simulink library "components_lib"  (Simulink 6.2)
undefined symbols (not defined in the file): A_ang_c, A_att_c, A_est, A_kalman, albedo_onboard_wrapper, B_ang_c, B_att_c, B_est, B_kalman, C_ang_c, C_att_c, C_est, C_i, C_kalman, C_p, Cd, D_ang_c, D_att_c, D_est, D_kalman, Dim, DiscIntNeverNeededParam, Hr, Hs, inerti, Ki, Kr, Ks, magnitude, otoquest, otoquest_with_pro, qmethod, rho, sat_temp_start, ss_proj3, sun_emu_angles2currents, sun_emu_vec2angles, Ts, vector_projection_onto_plane, w_mw_i, w_mw_init, zenith2ref
libraries: components_lib x163, simulink x44, albedo_lib x4, Accessories_lib x3, simulink_extras x2, discrete_bdot_filter x1
(part 1 of 5)
settings Model: Creator=jdgr01  LastModifiedBy=Martin  ExtModeAutoUpdateStatusClock=off

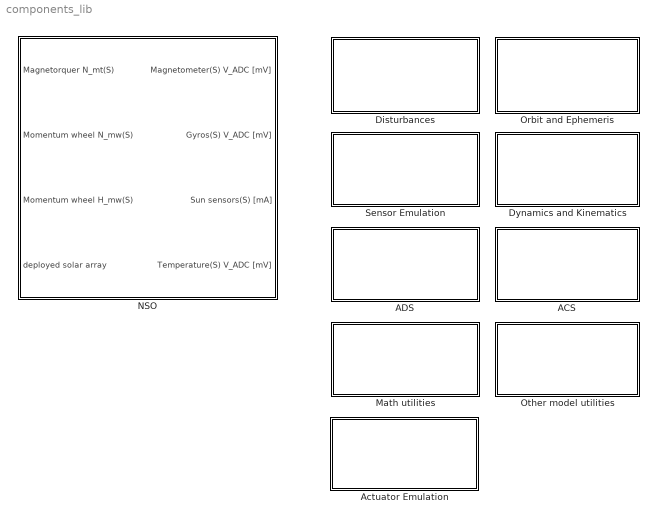
== system components_lib ==
  ACS : Subsystem
  ADS : Subsystem
  Actuator Emulation : Subsystem
  Disturbances : Subsystem
  Dynamics and Kinematics : Subsystem
  Math utilities : Subsystem
  NSO : Subsystem  Tag=AAUSAT-II Model  Description=AAUSAT-II Model  mask{r_com_s=[0.05 0.05 0.15], sat_temp_start=0, r_com_s_deployed=[0.05 0.05 0.125], mass_sc=3, Dim=[0.1 0.1 0.3], inertia_c=[25 25 5]/1e3, inertia_d=[42.3 42.3 28.4]/1e3, init_jd=2452315.56, q_s_c=[0 0 0 1], q_init_s_i=[sqrt(0.5) 0 0 sqrt(0.5)], w_init_s=[0.1 0.1 0.1]*0, Cd=2, rho=9.25e-13, enable_sensor_emulation=off, alb_emu_enabled=off, enable_dist=off}
      mask prompts: r_com_s "Center of mass (S)"; sat_temp_start "Start temperature of satellite [K]"; r_com_s_deployed "Center of mass (deployed)"; mass_sc "Mass of spacecraft (kg)"; Dim "Dimensions of the satellite (m)"; inertia_c "Folded inertia matrix(C)"; inertia_d "Deployed inertia matrix(C)"; init_jd "Initial time (JD)"; q_s_c "Controller reference frame (S->C)"; q_init_s_i "Initial attitude q_i(S->I)"; w_init_s "Initial angular rate W(S)"; Cd "Drag Coefficient"; rho "Air Density"; enable_sensor_emulation "Enable sensor emulation?"; alb_emu_enabled "Enable albedo emulation?"; enable_dist "Enable disturbances"
      mask Display:
      | image(imread('NSO.jpg'));
      | color('r');
      | port_label('input', 1, 'N_mt(S)');
      | port_label('input', 2, 'N_mw(S)');
      | port_label('input', 3, 'H_mw(S)');
      | port_label('input', 4, 'Deployed solar array');
      | port_label('output', 1, 'Magnetometer(S) V_ADC [mV]');
      | port_label('output', 2, 'Gyros(S) V_ADC [mV]');
      | port_label('output', 3, 'Sun sensors(S) [mA]');
      | port_label('output', 4, 'Temperature(S) V_ADC [mV]');
  Orbit and Ephemeris : Subsystem
  Other model utilities : Subsystem
  Sensor Emulation : Subsystem

== system components_lib/ACS ==
  Controllers : Subsystem
  Magnetorquer power driver : Subsystem
  magnetorquer driver : Subsystem
      mask Display:
      | port_label('output',1,'I_out')
      | port_label('input',1,'Nmt(sat)')
      | port_label('input',2,'B(sat)')

== system components_lib/ADS ==
  Attitude Determination : Subsystem
  FDI : Subsystem
  On-board model : Subsystem

== system components_lib/Actuator Emulation ==
  Magnetorquer : Subsystem  mask{v_max_mt=5, coil_dim=[0.07 0.21], L_mt=26.956e-3, n_mt=435, A_wire_mt=(pi/4)*0.0002^2, sigma_0_mt=1.7e-8, alpha_0_mt=3.9e-3, T_0_mt=293}
      mask prompts: v_max_mt "Maximum voltage"; coil_dim "Coil dimensions [x y]"; L_mt "Coil inductance"; n_mt "Coil winding number"; A_wire_mt "Wire cross sectional area"; sigma_0_mt "Wire resistivity"; alpha_0_mt "Wire resistivity temp. coef."; T_0_mt "Wire resistivity base temp."
  Magnetorquer without L : Subsystem  mask{v_max_mt=5, coil_dim=[0.07 0.21], n_mt=435, A_wire_mt=(pi/4)*0.0002^2, sigma_0_mt=1.7e-8, alpha_0_mt=3.9e-3, T_0_mt=293}
      mask prompts: v_max_mt "Maximum voltage"; coil_dim "Coil dimensions [x y]"; n_mt "Coil winding number"; A_wire_mt "Wire cross sectional area"; sigma_0_mt "Wire resistivity"; alpha_0_mt "Wire resistivity temp. coef."; T_0_mt "Wire resistivity base temp."
  Momentum wheel : Subsystem  mask{v_max_mw=3, v_min_mw=0, R_mw=8, L_mw=0.07e-3, C_t=2.67e-3, C_s=0.0027, mu_f=39.606e-9, I_mw=4.139e-6}
      mask prompts: v_max_mw "Maximum voltage"; v_min_mw "Minimum voltage"; R_mw "Amature resistance"; L_mw "Amature inductance"; C_t "Motor torque constant"; C_s "Motor speed constant"; mu_f "Viscous friction coef."; I_mw "Momentum wheel inertia"
  NSO magnetorquers : Subsystem
  NSO magnetorquers without L : Subsystem
  NSO momentum wheels : Subsystem  mask{w_mw_i=[1078.6 1078.6 1078.6] *0.5}
      mask prompts: w_mw_i "Initial Angular Velocity"
  NSO mw HW : Subsystem  mask{C_p=0.4, C_i=0.04, w_mw_init=w_mw_i(1)}
      mask prompts: C_p "Motor controller p-gain"; C_i "Motor controller i-gain"; w_mw_init "Initial Angular velocity"
  PI-controller : Subsystem  mask{PI_cp=C_p, PI_ci=C_i, int_limit_max=3, int_limit_min=-3}
      mask prompts: PI_cp "Porpotional gain"; PI_ci "Integrator gain"; int_limit_max "Integrator limit max"; int_limit_min "Integrator limit min"

== system components_lib/Disturbances ==
  Atmospheric : Subsystem
  Disturbances : Subsystem
  Exposed area : Subsystem  mask{dim_sat_area=Dim, dim_sat_array=[-0.30,-0.30]}
      mask prompts: dim_sat_area "Satellite Body Dimentions [x,y,z]"; dim_sat_array "Solar Array Dimentions [array1_y,array2_x]"
  Gravity : Subsystem  mask{G=6.673e-11, M_sun=1.98892e30, M_moon=7.36e22, M_earth=5.9742e24}
      mask prompts: G "Gravitational Constant (m^3/kgs^2)"; M_sun "Mass of the Sun (kg)"; M_moon "Mass of the Moon (kg)"; M_earth "Mass of the Earth (kg)"
  Magnetic residual disturbance : Subsystem
  Radiation (I) : Subsystem

== system components_lib/Dynamics and Kinematics ==
  Spacecraft Dynamics : Subsystem

== system components_lib/Math utilities ==
  Quaternion operations : Subsystem
  Vector operations : Subsystem

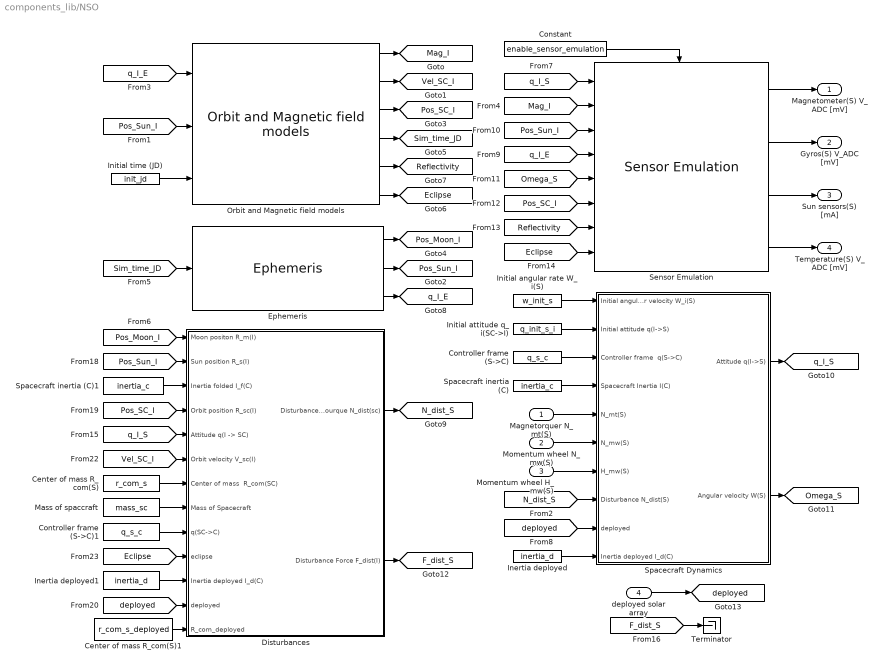
== system components_lib/NSO ==
  Magnetorquer N_mt(S) : Inport  Port=1  LatchInput=off
  Momentum wheel N_mw(S) : Inport  Port=2  LatchInput=off
  Momentum wheel H_mw(S) : Inport  Port=3  LatchInput=off
  deployed solar array : Inport  Port=4  LatchInput=off
  Center of mass R_com(S) : Constant  Value=r_com_s
  Center of mass R_com(S)1 : Constant  Value=r_com_s_deployed
  Constant : Constant  Value=enable_sensor_emulation
  Controller frame (S->C) : Constant  Value=q_s_c
  Controller frame (S->C)1 : Constant  Value=q_s_c
  Disturbances : Subsystem  AncestorBlock=components_lib/Disturbances/Disturbances
  Ephemeris : components_lib/Orbit and Ephemeris/Ephemeris
  Inertia deployed : Constant  Value=inertia_d
  Inertia deployed1 : Constant  Value=inertia_d
  Initial angular rate W_i(S) : Constant  Value=w_init_s
  Initial attitude q_i(SC->I) : Constant  Value=q_init_s_i
  Initial time (JD) : Constant  Value=init_jd
  Mass of spaccraft : Constant  Value=mass_sc
  Orbit and Magnetic field models : components_lib/Orbit and Ephemeris/Orbit and Magnetic field models  data_type=SGP4/IGRF models  tle_type=Oersted TLE  reflectivity_enabled=0
  Sensor Emulation : components_lib/Sensor Emulation/Sensor Emulation
  Spacecraft Dynamics : Subsystem  AncestorBlock=components_lib/Dynamics and Kinematics/Spacecraft Dynamics
  Spacecraft inertia (C) : Constant  Value=inertia_c
  Spacecraft inertia (C)1 : Constant  Value=inertia_c
  Terminator : Terminator
  Magnetometer(S) V_ADC [mV] : Outport
  Gyros(S) V_ADC [mV] : Outport  Port=2
  Sun sensors(S) [mA] : Outport  Port=3
  Temperature(S) V_ADC [mV] : Outport  Port=4
  tag scope: Eclipse=global, F_dist_S=global, Mag_I=global, N_dist_S=global, Omega_S=global, Pos_Moon_I=global, Pos_SC_I=global, Pos_Sun_I=global, Reflectivity=global, Sim_time_JD=global, Vel_SC_I=global, deployed=global, q_I_E=global, q_I_S=global
  wires:
  [N_dist_S] -> Spacecraft Dynamics/8(Disturbance N_dist(S))
  Center of mass R_com(S)1/1 -> Disturbances/13(R_com_deployed)
  Momentum wheel N_mw(S)/1 -> Spacecraft Dynamics/6(N_mw(S))
  [Eclipse] -> Disturbances/10(eclipse)
  [Reflectivity] -> Sensor Emulation/7
  [Pos_SC_I] -> Sensor Emulation/6
  [Omega_S] -> Sensor Emulation/5
  [q_I_E] -> Sensor Emulation/4
  [Mag_I] -> Sensor Emulation/2
  [Pos_Sun_I] -> Sensor Emulation/3
  [q_I_S] -> Sensor Emulation/1
  [Vel_SC_I] -> Disturbances/6(Orbit velocity V_sc(I))
  [q_I_S] -> Disturbances/5("Attitude q(I -> SC)")
  [Pos_SC_I] -> Disturbances/4(Orbit position R_sc(I))
  Initial time (JD)/1 -> Orbit and Magnetic field models/3
  [Pos_Sun_I] -> Disturbances/2(Sun position R_s(I))
  [Pos_Moon_I] -> Disturbances/1(Moon positon R_m(I))
  [Pos_Sun_I] -> Orbit and Magnetic field models/2
  [Sim_time_JD] -> Ephemeris/1
  Spacecraft Dynamics/2(Angular velocity W(S)) -> [Omega_S]
  Spacecraft Dynamics/1(Attitude q(I->S)) -> [q_I_S]
  Disturbances/2(Disturbance Force F_dist(I)) -> [F_dist_S]
  Orbit and Magnetic field models/5 -> [Reflectivity]
  Ephemeris/3 -> [q_I_E]
  Ephemeris/2 -> [Pos_Sun_I]
  Ephemeris/1 -> [Pos_Moon_I]
  Orbit and Magnetic field models/4 -> [Sim_time_JD]
  Initial attitude q_i(SC->I)/1 -> Spacecraft Dynamics/2(Initial attitude q(I->S))
  Initial angular rate W_i(S)/1 -> Spacecraft Dynamics/1(Initial angular velocity W_i(S))
  Orbit and Magnetic field models/3 -> [Pos_SC_I]
  Controller frame (S->C)/1 -> Spacecraft Dynamics/3(Controller frame  q(S->C))
  Spacecraft inertia (C)/1 -> Spacecraft Dynamics/4(Spacecraft Inertia I(C))
  Spacecraft inertia (C)1/1 -> Disturbances/3(Inertia folded I_f(C))
  Center of mass R_com(S)/1 -> Disturbances/7(Center of mass  R_com(SC))
  [q_I_E] -> Orbit and Magnetic field models/1
  Orbit and Magnetic field models/2 -> [Vel_SC_I]
  Sensor Emulation/3 -> Sun sensors(S) [mA]/1
  Sensor Emulation/2 -> Gyros(S) V_ADC [mV]/1
  Sensor Emulation/1 -> Magnetometer(S) V_ADC [mV]/1
  Orbit and Magnetic field models/1 -> [Mag_I]
  Mass of spaccraft/1 -> Disturbances/8("Mass of Spacecraft ")
  Controller frame (S->C)1/1 -> Disturbances/9(q(SC->C))
  Momentum wheel H_mw(S)/1 -> Spacecraft Dynamics/7(H_mw(S))
  Magnetorquer N_mt(S)/1 -> Spacecraft Dynamics/5(N_mt(S))
  Sensor Emulation/4 -> Temperature(S) V_ADC [mV]/1
  Orbit and Magnetic field models/6 -> [Eclipse]
  [Eclipse] -> Sensor Emulation/8
  [F_dist_S] -> Terminator/1
  deployed solar array/1 -> [deployed]
  Inertia deployed/1 -> Spacecraft Dynamics/10(Inertia deployed I_d(C))
  [deployed] -> Spacecraft Dynamics/9(deployed)
  [deployed] -> Disturbances/12(deployed)
  Inertia deployed1/1 -> Disturbances/11(Inertia deployed I_d(C))
  Disturbances/1(Disturbance tourque N_dist(sc)) -> [N_dist_S]
  Constant/1 -> Sensor Emulation/Enable

== system components_lib/Orbit and Ephemeris ==
  (IGRF) Magnetic field : Subsystem  TreatAsAtomicUnit=on
  Albedo : Subsystem  TreatAsAtomicUnit=on
  Albedo emulation model : Subsystem
  Eclipse model : Subsystem  mask{r_e=6371010, theta_e=65}
      mask prompts: r_e "Radius of Earth [m]"; theta_e "Max. angle of theta [deg] (eclipse: theta > r_earth/norm(R_SA))"
      mask Display:
      | image(imread('eclipse.jpg'));
      | color('white');
      | port_label('input', 1, 'Sun vector (I)');
      | port_label('input', 2, 'Satellite vector (I)');
      | port_label('output', 1, 'Eclipse');
      | fprintf('1=true,\n 0=false')
  Ephemeris : Subsystem
  Magnetic field model : Subsystem
  Orbit and Magnetic field models : Subsystem  mask{data_type=SGP4/IGRF models, tle_type=Oersted TLE, reflectivity_enabled=0}
      mask prompts: data_type "Data to use for Pos. and mag. field"; tle_type "Choose which TLE to use for SGP4"; reflectivity_enabled "Calculate reflectivity matrix"
      mask help: When you want to use "Other" make sure to define the TLE in the SGP4 subsystem.
      mask init:
      | % if oersted data -> data_type=1
      | % if SGP4/IGRF model -> data_type=2
      | 
      | disp('Using Oersted data for Pos./mag field. Loading measurement data...');
      | load('oersted_data.mat')
      | 
      | if data_type==1
      |     disp('Done loading Oersted data...');
      |     enable_oersted=1;
      |     enable_sgp4 = 0;
      |     enable_IGRF = 0;
      |     enable_custom_time = 0;
      | else
      |     disp('Using SGP4/IGRF model for Pos./mag field.');
      |     enable_oersted = 0;
      |     enable_sgp4 = 1;
      |     enable_IGRF = 1;
      |     enable_custom_time = 1;
      | end
      | 
      | if tle_type==1 %Choose which TLE to use
      |     enable_oersted_tle=1;
      |     enable_other_tle=0;
      | else
      |     enable_oersted_tle=0;
      |     enable_other_tle=1;
      | end
      mask StyleString: popup(Oersted meas data|SGP4/IGRF models),popup(Oersted TLE|Other TLE),edit

== system components_lib/Other model utilities ==
  AAUSAT-II Animation : Subsystem  mask(AAUSAT-II Animation){u1=[-20000000 20000000 -20000000 20000000 -20000000 20000000], u2=50, u3=1000000, u20=on, u18=15, u4=6378000, u11=80, u12=on, u13='earth280.jpg', u17=180, u5=Fixed position, u6=[70000000 70000000 70000000], u7=8, u9=off, u10=on, u16=off, u14=on, u15=on, u8=on, u19=off}
      mask prompts: u1 "Axes limits [xmin xmax ymin ymax zmin zmax]:"; u2 "Time interval between updates:"; u3 "Size of spacecraft displayed:"; u20 "Use spacecraft image map"; u18 "Spacecraft drawing slices"; u4 "Planet radius:"; u11 "Planet drawing slices"; u12 "Use planet map"; u13 "Planet map image file"; u17 "Pre-rotate image map (deg)"; u5 "Enter view:"; u6 "Position of camera [xc yc zc]:"; u7 "View angle:"; u9 "Show SC coordinate system"; u10 "Show orbit coordinate system"; u16 "Show Earth Centered Earth Fixed coordinate system"; u14 "Show inertial coordinate system"; u15 "Show trajectory"; u8 "Enable animation"; u19 "Make movie (use with care!)"
      mask help:
      | Create a 3-D animated view of the AAUSAT-II, where X, Y, and Z craft position (Position) and craft quaternion (Attitude) are inputs.
      |
      | Display parameters are in the same units of length as the input parameters.
      |
      | Created by Karl Laursen
      mask init:
      | Config.axes = u1;
      | Config.update = u2;
      | Config.craft = u3;
      | Config.radius = u4;
      | Config.camera_view = u5;
      | Config.camera_pos = u6;
      | Config.view = u7;
      | Config.Animenable = u8;
      | Config.ShowSCFrame = u9;
      | Config.ShowOrbitFrame = u10;
      | Config.ShowECEF = u16;
      | Config.ShowInertial = u14;
      | Config.PlanetSlices = u11;
      | Config.UseMap = u12;
      | Config.PlanetMapFile = u13;
      | Config.Trajectory = u15;
      | Config.PreRotation = u17;
      | Config.CraftSlices = u18;
      | Config.MakeMovie = u19;
      | Config.UseSCMap = u20;
      mask Help: web(asbhelp('6dofanimation'));
      mask StyleString: edit,edit,edit,checkbox,edit,edit,edit,checkbox,edit,edit,popup(Fixed position|Fly alongside),edit,edit,checkbox,checkbox,checkbox,checkbox,checkbox,checkbox,checkbox

== system components_lib/Sensor Emulation ==
  Emulation of gyros : Subsystem  mask(Parameters for the gyro sensor block){scale_model=[859.4 859.4 859.4 859.4 859.4 859.4], offset_model=[2500 2500 2500 2500 2500 2500], e_bias=[0.0012 0.0012 0.0012 0.0012 0.0012 0.0012], e_align=[1 1 1 1 1 1], e_scale=[0.1 0.1 0.1 0.1 0.1 0.1], e_noise=[0.0035 0.0035 0.0035 0.0035 0.0035 0.0035]*1e-6, e_noise_seed=[23341 43534 43433 22299 32478 21932], e_drift_scale_model=[0.075 0.075 0.075 0.075 0.075 0.075], e_drift_offset_model=[0.012 0.012 0.012 0.012 0.012 0.012], op_amp_gain=[10 10 10 10 10 10], op_amp_offset=[2500 2500 2500 2500 2500 2500]}
      mask prompts: scale_model "Gyro model: Scale factor (mV/rad/s)"; offset_model "Gyro model: Offset (mV)"; e_bias "Gyro model: Bias (rad/s)"; e_align "Gyro model: Misalignment (degree)"; e_scale "Gyro model: Scale error (%)"; e_noise "Gyro model: Standard deviation"; e_noise_seed "Gyro model: Noise randomizer seed"; e_drift_scale_model "Gyro model: Scale factor drift (%/K)"; e_drift_offset_model "Gyro model: Offset drift (rad/s/K)"; op_amp_gain "Amplification HW: Op-amp gain ()"; op_amp_offset "Amplification HW: Op-amp offset (mV)"
      mask help:
      | Fill out the parameters for use in the simulation.
      | format of the parameter field: (gyro1 gyro2 gyro3 gyro4 gyro5 gyro6)
      | gyro 1 and gyro 4 are situated on the same axis, but in opposite directions etc.
      mask init:
      | e_align_coor_factor=gyroalign(e_align);
  Emulation of magnetometer : Subsystem  mask{v_supply_model=5, sens_model=[1 1 1], e_drift_sens_model=[-3000 -3000 -3000], e_scale=[0.05 0.05 0.05], e_align=1*0, e_orth=1*0, e_noise=[32 32 32]*1e-6*0, e_noise_seed=[23341 43534 43433], op_amp_gain=[500 500 500], op_amp_offset=[2500 2500 2500]}
      mask prompts: v_supply_model "Magnetometer model: Supply voltage (V)"; sens_model "Magnetometer model: Sensitivity (mV/V/gauss)"; e_drift_sens_model "Magnetometer model: Sensitivity drift due to temperature (ppm/K)"; e_scale "Magnetometer model: Scale error (%)"; e_align "Magnetometer model: Missalignment (degree) - Only one value!"; e_orth "Magnetometer model: Orthogonality error (degree) - Only one value!"; e_noise "Magnetometer model: Noise,standard deviation"; e_noise_seed "Magnetometer model: Noise randomizer seed ()"; op_amp_gain "Amplification HW: Op-amp gain ()"; op_amp_offset "Amplification HW: Op-amp offset (mV)"
      mask init:
      | e_align_coor_factor=magalign(e_align+e_orth);
  Emulation of temperature sensors : Subsystem
  Sensor Emulation : Subsystem
  Sun sensors : Subsystem  mask{sun_flux=1366.9, alpha_align=[1 1 1 1 2 2]*0, temp_drift=0.00233, sigma_noise=0.0000014*0, noise_seed=[0.0000008 0.0000011 0.0000004 0.0000005 0.0000000 0.0000002]*0, op_amp_gain=1, op_amp_offset=0}
      mask prompts: sun_flux "Sun sensor model: Solar Flux"; alpha_align "Sun sensor model: Alignment error vector (x+,y+,z+,x-,y-,z-)"; temp_drift "Sun sensor model: Temperature dependence"; sigma_noise "Sun sensor model: Noise standard deviation"; noise_seed "Sun sensor model: Noise seed"; op_amp_gain "Sensor signal amplification: Gain"; op_amp_offset "Sensor signal amplification: Offset"
      mask init:
      | angle2current_model = sun_emu_model();
      | i_dark = polyval(angle2current_model, 90);
      | i_max = polyval(angle2current_model, 0);

== system components_lib/ACS/Controllers ==
  Angular velocity  controller : Subsystem  mask(Angular Velocity Controller){ang_file_name='ang_robust_control.m'}
      mask prompts: ang_file_name "Angular rate controller design file name (remember gnyfs :-))"
      mask help:
      | The controller in this block is to be constructed using a state space system. The
      | reference is subtracted from the measurement (positive feedback and SS-reference) and passed through the SS-system. Thus if the controller is merely a gain matrix only the D-matrix has to contain the controller and the remaining be zero-matrices. The controller design files are kept in the "design" directory and the definition of the controller system matrices is the final task in each controller design file.
      | The different matrices for the state space system are named:
      | A_ang_c
      | B_ang_c
      | C_ang_c
      | D_ang_c
      mask init:
      | run(strcat('design/',ang_file_name))
  Attitude controller : Subsystem  mask(Attitude Controller){att_file_name='attitude_control_lqr.m'}
      mask prompts: att_file_name "Attitude controller design file name (remember gnyfs :-))"
      mask help:
      | The controller in this block is to be constructed using a state space system. The error quarternion is calculated from the input and the result is used in the SS-system. Thus if the controller is merely a gain matrix only the D-matrix has to contain the controller and the remaining be zero-matrices. The controller design files are kept in the "design" directory and the definition of the controller system matrices is the final task in each controller design file.
      | The different matrices for the state space system are named:
      | A_att_c
      | B_att_c
      | C_att_c
      | D_att_c
      mask init:
      | run(strcat('design/',att_file_name))
  Attitude controller with integrator : Subsystem  mask(Attitude Controller){att_file_name='att_control_with_integrator.m'}
      mask prompts: att_file_name "Attitude controller design file name (remember gnyfs :-))"
      mask help:
      | The controller in this block is to be constructed using a state space system. The error quarternion is calculated from the input and the result is used in the SS-system. Thus if the controller is merely a gain matrix only the D-matrix has to contain the controller and the remaining be zero-matrices. The controller design files are kept in the "design" directory and the definition of the controller system matrices is the final task in each controller design file.
      | The different matrices for the state space system are named:
      | A_att_c
      | B_att_c
      | C_att_c
      | D_att_c
      mask init:
      | run(strcat('design/',att_file_name))
  Desaturation controller : Subsystem  mask{h_bias=2.23*1e-3}
      mask prompts: h_bias "Angular momentum bias"
  Detumble controller : Subsystem  Orientation=left  mask{C_cont=11000, w_c=0.7, C_disc=1500, ctrl=none}
      mask prompts: C_cont "B-dot continous gain"; w_c "B-dot filter cut-off frequency"; C_disc "B-dot discrete gain"; ctrl "Controller"
      mask StyleString: edit,edit,edit,popup(none|Continous|Discrete)
  Estimation of dist Kalman filter : Subsystem  mask(Estimator Block){ang_file_name='kalman_estimator.m'}
      mask prompts: ang_file_name "Estimator design file name (remember gnyfs :-))"
      mask help:
      | The estimator in this block is to be constructed using a state space system.
      | The estimator block has three input (the control torque, measured quaternion and measured angular velocity).
      | The design of the estimator is developed in an m-file located in the design folder
      | The different matrices for the state space system are named:
      | A_kalman
      | B_kalman
      | C_kalman
      | D_kalman
      mask init:
      | run(strcat('design/',ang_file_name))
  Estimation of dist linear filter : Subsystem  mask(Estimator Block){ang_file_name='linear_estimator.m'}
      mask prompts: ang_file_name "Estimator design file name (remember gnyfs :-))"
      mask help:
      | The estimator in this block is to be constructed using a state space system.
      | The estimator block has three input (the control torque, measured quaternion and measured angular velocity).
      | The design of the estimator is developed in an m-file located in the design folder
      | The different matrices for the state space system are named:
      | A_est
      | B_est
      | C_est
      | D_est
      mask init:
      | run(strcat('design/',ang_file_name))
  LQ-Regulator : Subsystem

== system components_lib/ACS/Magnetorquer power driver ==
  m_mt(S) : Inport  Port=1  LatchInput=off
  Demux : Demux  Outputs=3
  Gain : Gain  Gain=0.408163
  Gain1 : Gain  Gain=0.408163
  Gain2 : Gain  Gain=0.408163
  Mux : Mux  Inputs=3
  I out : Outport
  wires:
  Demux/3 -> Gain2/1
  Demux/2 -> Gain1/1
  Demux/1 -> Gain/1
  m_mt(S)/1 -> Demux/1
  Mux/1 -> I out/1
  Gain1/1 -> Mux/2
  Gain/1 -> Mux/1
  Gain2/1 -> Mux/3

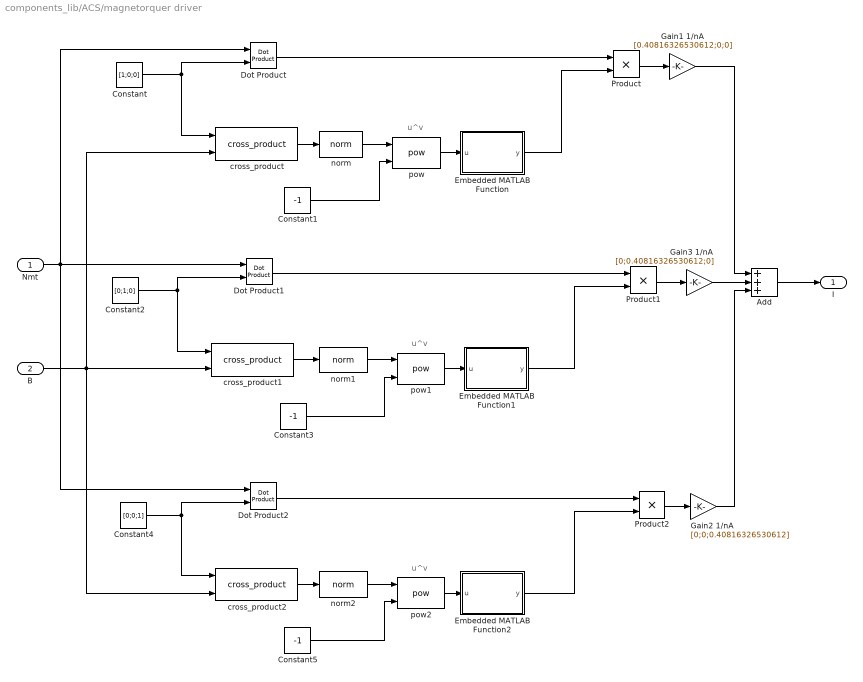
== system components_lib/ACS/magnetorquer driver ==
  note: u^v
  note: u^v
  note: u^v
  Nmt : Inport  Port=1  LatchInput=off
  B : Inport  Port=2  LatchInput=off
  Add : Sum  Inputs=+++  OutScaling=2^-10
  Constant : Constant  Value=[1;0;0]
  Constant1 : Constant  Value=-1
  Constant2 : Constant  Value=[0;1;0]
  Constant3 : Constant  Value=-1
  Constant4 : Constant  Value=[0;0;1]
  Constant5 : Constant  Value=-1
  Dot Product : simulink/Math Operations/Dot Product  InputSameDT=on  OutDataType=sfix(16)  OutScaling=2^-10  DoSatur=off
  Dot Product1 : simulink/Math Operations/Dot Product  InputSameDT=on  OutDataType=sfix(16)  OutScaling=2^-10  DoSatur=off
  Dot Product2 : simulink/Math Operations/Dot Product  InputSameDT=on  OutDataType=sfix(16)  OutScaling=2^-10  DoSatur=off
  Embedded MATLAB Function : Stateflow chart
  Embedded MATLAB Function1 : Stateflow chart
  Embedded MATLAB Function2 : Stateflow chart
  Gain1 1/nA : Gain  Gain=[0.40816326530612;0;0]
  Gain2 1/nA : Gain  Gain=[0;0;0.40816326530612]
  Gain3 1/nA : Gain  Gain=[0;0.40816326530612;0]
  Product : Product  RndMeth=Zero
  Product1 : Product  RndMeth=Zero
  Product2 : Product  RndMeth=Zero
  cross_product : components_lib/Math utilities/Vector operations/cross_product
  cross_product1 : components_lib/Math utilities/Vector operations/cross_product
  cross_product2 : components_lib/Math utilities/Vector operations/cross_product
  norm : components_lib/Math utilities/Vector operations/norm
  norm1 : components_lib/Math utilities/Vector operations/norm
  norm2 : components_lib/Math utilities/Vector operations/norm
  pow : components_lib/Math utilities/Vector operations/pow  Description=u^v
  pow1 : components_lib/Math utilities/Vector operations/pow  Description=u^v
  pow2 : components_lib/Math utilities/Vector operations/pow  Description=u^v
  I : Outport
  wires:
  B/1 -> cross_product2/2, cross_product/2, cross_product1/2
  Nmt/1 -> Dot Product2/1, Dot Product/1, Dot Product1/1
  Embedded MATLAB Function2/1(y) -> Product2/2
  pow2/1 -> Embedded MATLAB Function2/1(u)
  Embedded MATLAB Function1/1(y) -> Product1/2
  pow1/1 -> Embedded MATLAB Function1/1(u)
  Embedded MATLAB Function/1(y) -> Product/2
  pow/1 -> Embedded MATLAB Function/1(u)
  Gain2 1/nA/1 -> Add/3
  Constant/1 -> cross_product/1, Dot Product/2
  Dot Product/1 -> Product/1
  Product/1 -> Gain1 1/nA/1
  Constant1/1 -> pow/2
  cross_product/1 -> norm/1
  norm/1 -> pow/1
  Constant2/1 -> cross_product1/1, Dot Product1/2
  Dot Product1/1 -> Product1/1
  Product1/1 -> Gain3 1/nA/1
  Constant3/1 -> pow1/2
  cross_product1/1 -> norm1/1
  norm1/1 -> pow1/1
  Constant4/1 -> cross_product2/1, Dot Product2/2
  Dot Product2/1 -> Product2/1
  Product2/1 -> Gain2 1/nA/1
  Constant5/1 -> pow2/2
  cross_product2/1 -> norm2/1
  norm2/1 -> pow2/1
  Gain3 1/nA/1 -> Add/2
  Gain1 1/nA/1 -> Add/1
  Add/1 -> I/1

== system components_lib/ADS/Attitude Determination ==
  EKF using quaternions : Subsystem
  EKF using sun and mag vectors : Subsystem
  EKF using sun and mag vectors .. and removing bias : Subsystem
  Propagator from Kalman filter : Subsystem
  otoquest : Subsystem
  otoquest with propagator : Subsystem
  q-method : Subsystem

== system components_lib/ADS/FDI ==
  Residual Generator : Subsystem  mask{poles=[10,10,10,10,10,10,10,10,10,10], h_mw=[0;0;0], w_bar=[0;0;0], q_bar=[0;0;0;0], I=eye(3), Q=eye(10), S_w=0, S_Iw=0, S_hm=0, A=0, B=0, C=0, L=0}
      mask prompts: poles "Observer Poles"; h_mw "momentum wheel working point"; w_bar "omega working point"; q_bar "attitude working point"; I "Inertia Matrix"; Q "Residual Matrix (Q)"; S_w "Skew symetric omega"; S_Iw "Skew symetric Iw"; S_hm "Skew symetric momentum wheel"; A "System Matrix"; B "Input Matrix"; C "Output Matrix"; L "Observer Matrix"
      mask init:
      | S_w = [0 -w_bar(3) w_bar(2);w_bar(3) 0 -w_bar(1);-w_bar(2) w_bar(1) 0];
      | S_mw = [0 -h_mw(3) h_mw(2);h_mw(3) 0 -h_mw(1);-h_mw(2) h_mw(1) 0];
      | S_Iw = [0 -w_bar(3)*I(3) w_bar(2)*I(2);w_bar(3)*I(3) 0 -w_bar(1)*I(1);-w_bar(2)*I(2) w_bar(1)*I(1) 0];
      | A = [-S_w, zeros(3,1), 0.5*eye(3), zeros(3,3);zeros(1,10);zeros(3,4), inv(I)*(S_Iw - S_w*I + S_mw), -inv(I)*S_w;zeros(3,10)];
      | B = [zeros(4,3) zeros(4,3);inv(I),-inv(I);zeros(3,3), eye(3)];
      | C = eye(10);
      | L = place(A',C',-poles);

== system components_lib/ADS/On-board model ==
  ADS on-board models : Subsystem  mask{sun_flux=1366.9, alb_enabled=off}
      mask prompts: sun_flux "Solar flux [W/m^2]"; alb_enabled "Albedo enabled"
  Albedo emulation model : Subsystem
  Albedo model onboard : Subsystem  mask{sun_flux=1366.9, matrix=FOV cosine dep. reflectivity table, enable=off}
      mask prompts: sun_flux "Sun flux (mean: 1366.9)"; matrix "Choose used reflectivity data:"; enable "Use reflectivity matrix (blackbox)"
      mask init:
      | if matrix == 1
      |     mrm = load('fov_albedo_matrix.mat');
      |     mrm = mrm.mrm;  
      | elseif matrix == 2
      |     mrm = load('fov_meaned_albedo_matrix.mat');
      |     mrm = mrm.mrm;
      | elseif matrix == 3
      |     mrm = load('fov_albedo_polynomial_matrix.mat');
      |     mrm = mrm.mrm;
      | elseif matrix == 4
      |     mrm = ones(180,288).*0.30;
      | end
      mask StyleString: edit,popup(FOV cosine dep. reflectivity table|FOV meaned reflectivity table|Polynomial fit to latitude meaned reflectivity|Constant reflectivity of 30%),checkbox
  Albedo projection : Subsystem
  Eclipse model : Subsystem  mask{r_e=6371010, theta_e=65}
      mask prompts: r_e "Radius of Earth [m]"; theta_e "Max. angle of theta [deg] (eclipse: theta > r_earth/norm(R_SA))"
      mask Display:
      | image(imread('eclipse.jpg'));
      | color('white');
      | port_label('input', 1, 'Sun vector (I)');
      | port_label('input', 2, 'Satellite vector (I)');
      | port_label('output', 1, 'Eclipse');
      | fprintf('1=true,\n 0=false')
  Ephemeris on-board : Subsystem
  Gyros : Subsystem  mask(Parameters for the gyro sensor block){op_amp_gain=[10 10 10 10 10 10], op_amp_offset=[2500 2500 2500 2500 2500 2500], scale_obc_alg=[859.4 859.4 859.4 859.4 859.4 859.4 ], offset_obc_alg=[2500 2500 2500 2500 2500 2500], e_drift_scale_obc_alg=[0.075 0.075 0.075 0.075 0.075 0.075], e_drift_offset_obc_alg=[10 10 10 10 10 10]}
      mask prompts: op_amp_gain "Amplification HW: Op-amp gain ()"; op_amp_offset "Amplification HW: Op-amp offset (mV)"; scale_obc_alg "OBC algorithms: Scale factor (mV/rad/s)"; offset_obc_alg "OBC algorithms: offset (mV)"; e_drift_scale_obc_alg "OBC algorithms: Scale factor drift (%/K)"; e_drift_offset_obc_alg "OBC algorithms: Offset drift (mV/K)"
      mask help:
      | Fill out the parameters for use in the simulation.
      | format of the parameter field: (gyro1 gyro2 gyro3 gyro4 gyro5 gyro6)
      | gyro 1 and gyro 4 are situated on the same axis, but in opposite directions etc.
  Magnetic field model : Subsystem
  Magnetometer : Subsystem  mask{op_amp_gain=[500 500 500], v_supply_model=5, op_amp_offset=[2500 2500 2500], sens_obc_alg=[1 1 1], e_drift_sens_obc_alg=[-3000 -3000 -3000], e_offset_obc_alg=[10 10 10]*0}
      mask prompts: op_amp_gain "Amplification HW: Op-amp gain ()"; v_supply_model "Magnetometer supply voltage (V)"; op_amp_offset "Amplification HW: Op-amp offset (mV)"; sens_obc_alg "OBC algorithms: Sensitivity (mV/V/gauss)"; e_drift_sens_obc_alg "OBC algorithms: Sensitivity drift due to temperature (ppm/K)"; e_offset_obc_alg "OBC algorithms: offset (mV)"
  Orbit and Magnetic field models : Subsystem  mask{tle_type=Oersted TLE}
      mask prompts: tle_type "Choose which TLE to use for SGP4"
      mask help: When you want to use "Other" make sure to define the TLE in the SGP4 subsystem.
      mask init:
      | if tle_type==1 %Choose which TLE to use
      |     enable_oersted_tle=1;
      |     enable_other_tle=0;
      | else
      |     enable_oersted_tle=0;
      |     enable_other_tle=1;
      | end
      mask StyleString: popup(Oersted TLE|Other TLE)
  Sun sensors : Subsystem  mask{op_amp_gain=1, op_amp_offset=0, temp_drift=0.00233, I_dark=[0.0815 0.0815 0.0815 0.0815 0.0815 0.0815 ], I_max=[1.3928 1.3928 1.3928 1.3928 1.3928 1.3928]}
      mask prompts: op_amp_gain "Signal attenuation: Gain"; op_amp_offset "Signal attenuation: Offset"; temp_drift "Temperature drift compensation factor"; I_dark "Dark current compensation: Dark currents vector"; I_max "Current nomalization: Max currents vector"
      mask Display:
      | image(imread('sun.jpg'));
      | color('w');
      | port_label('input', 1, 'I_ADC[mA]');
      | port_label('input', 2, 'Temperature [K]');
      | port_label('output', 1, 'Sun position (s)');
  Temperature: Convert voltage from ADC into measured temperature : Subsystem
  sensor model : Subsystem

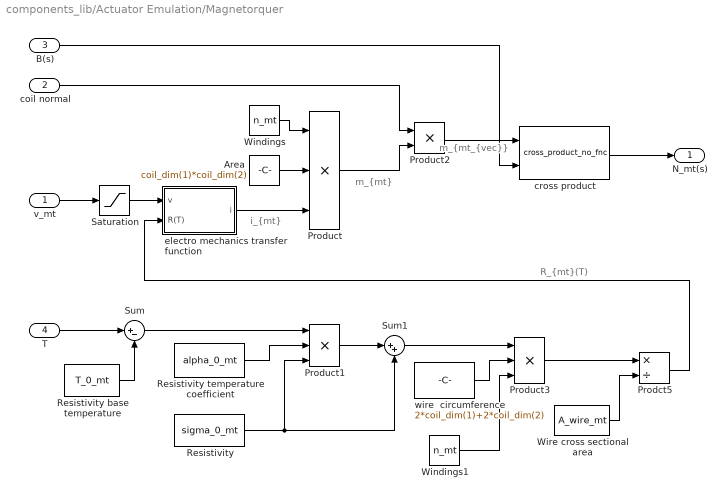
== system components_lib/Actuator Emulation/Magnetorquer ==
  note: R_{mt}(T)
  note: i_{mt}
  note: m_{mt}
  note: m_{mt_{vec}}
  v_mt : Inport  Port=1  LatchInput=off
  coil normal : Inport  Port=2  LatchInput=off
  B(s) : Inport  Port=3  LatchInput=off
  T : Inport  Port=4  LatchInput=off
  Area : Constant  Value=coil_dim(1)*coil_dim(2)
  Prodct5 : Product  Inputs=*/  RndMeth=Zero
  Product : Product  Inputs=3  RndMeth=Zero
  Product1 : Product  Inputs=3  RndMeth=Zero
  Product2 : Product  RndMeth=Zero
  Product3 : Product  Inputs=3  RndMeth=Zero
  Resistivity : Constant  Value=sigma_0_mt
  Resistivity base temperature : Constant  Value=T_0_mt
  Resistivity temperature coefficient : Constant  Value=alpha_0_mt
  Saturation : Saturate  UpperLimit=v_max_mt  LowerLimit=-v_max_mt
  Sum : Sum  Inputs=|+-
  Sum1 : Sum  Inputs=|++
  Windings : Constant  Value=n_mt
  Windings1 : Constant  Value=n_mt
  Wire cross sectional area : Constant  Value=A_wire_mt
  cross product : components_lib/Math utilities/Vector operations/cross_product_no_fnc
  electro mechanics transfer function : Subsystem
  wire  circumference : Constant  Value=2*coil_dim(1)+2*coil_dim(2)
  N_mt(s) : Outport
  wires:
  B(s)/1 -> cross product/2
  Prodct5/1 -> electro mechanics transfer function/2(R(T))
  Wire cross sectional area/1 -> Prodct5/2
  Product3/1 -> Prodct5/1
  Windings1/1 -> Product3/3
  wire  circumference/1 -> Product3/2
  Sum1/1 -> Product3/1
  Product1/1 -> Sum1/1
  Resistivity/1 -> Sum1/2, Product1/3
  Sum/1 -> Product1/1
  Resistivity temperature coefficient/1 -> Product1/2
  T/1 -> Sum/1
  Resistivity base temperature/1 -> Sum/2
  coil normal/1 -> Product2/1
  v_mt/1 -> Saturation/1
  Saturation/1 -> electro mechanics transfer function/1(v)
  electro mechanics transfer function/1(i) -> Product/3
  Windings/1 -> Product/1
  Area/1 -> Product/2
  Product/1 -> Product2/2
  Product2/1 -> cross product/1
  cross product/1 -> N_mt(s)/1

== system components_lib/Actuator Emulation/Magnetorquer without L ==
  note: m_{mt_{vec}}
  note: m_{mt}
  note: i_{mt}
  note: R_{mt}(T)
  v_mt : Inport  Port=1  LatchInput=off
  coil normal : Inport  Port=2  LatchInput=off
  B(s) : Inport  Port=3  LatchInput=off
  T : Inport  Port=4  LatchInput=off
  Area : Constant  Value=coil_dim(1)*coil_dim(2)
  Divide : Product  Inputs=*/  OutScaling=2^-10
  Prodct5 : Product  Inputs=*/  RndMeth=Zero
  Product : Product  Inputs=3  RndMeth=Zero
  Product1 : Product  Inputs=3  RndMeth=Zero
  Product2 : Product  RndMeth=Zero
  Product3 : Product  Inputs=3  RndMeth=Zero
  Resistivity : Constant  Value=sigma_0_mt
  Resistivity base temperature : Constant  Value=T_0_mt
  Resistivity temperature coefficient : Constant  Value=alpha_0_mt
  Saturation : Saturate  UpperLimit=v_max_mt  LowerLimit=-v_max_mt
  Sum : Sum  Inputs=|+-
  Sum1 : Sum  Inputs=|++
  Windings : Constant  Value=n_mt
  Windings1 : Constant  Value=n_mt
  Wire cross sectional area : Constant  Value=A_wire_mt
  cross product : components_lib/Math utilities/Vector operations/cross_product_no_fnc
  wire  circumference : Constant  Value=2*coil_dim(1)+2*coil_dim(2)
  N_mt(s) : Outport
  wires:
  B(s)/1 -> cross product/2
  cross product/1 -> N_mt(s)/1
  Product2/1 -> cross product/1
  Product/1 -> Product2/2
  Area/1 -> Product/2
  Windings/1 -> Product/1
  Divide/1 -> Product/3
  Saturation/1 -> Divide/1
  v_mt/1 -> Saturation/1
  coil normal/1 -> Product2/1
  Resistivity base temperature/1 -> Sum/2
  T/1 -> Sum/1
  Resistivity temperature coefficient/1 -> Product1/2
  Sum/1 -> Product1/1
  Resistivity/1 -> Product1/3, Sum1/2
  Product1/1 -> Sum1/1
  Sum1/1 -> Product3/1
  wire  circumference/1 -> Product3/2
  Windings1/1 -> Product3/3
  Product3/1 -> Prodct5/1
  Wire cross sectional area/1 -> Prodct5/2
  Prodct5/1 -> Divide/2

== system components_lib/Actuator Emulation/Momentum wheel ==
  note: e_{mw}
  note: i_{mw}
  note: N_{mw}
  note: \omega_{mw}
  V_mw : Inport  Port=1  LatchInput=off
  Bias1 : Constant  Value=I_mw
  Derivative : Derivative
  Electrical TF : TransferFcn  Denominator=[R_mw]
  Mechanical TF : Subsystem
  Motor speed  constant : Gain  Orientation=left  Gain=C_s
  Motor torque  constant : Gain  Gain=C_t
  Product : Product  RndMeth=Zero
  Product1 : Product  RndMeth=Zero
  Sum : Sum  Inputs=|+-
  Voltage  saturation : Saturate  UpperLimit=v_max_mw  LowerLimit=v_min_mw
  omega_mw : Outport
  N_mw : Outport  Port=2
  H_mw : Outport  Port=3
  wires:
  V_mw/1 -> Voltage  saturation/1
  Motor speed  constant/1 -> Sum/2
  Mechanical TF/1(w_mw) -> Motor speed  constant/1, Product/2, omega_mw/1, Product1/1
  Motor torque  constant/1 -> Mechanical TF/1(N_mw)
  Sum/1 -> Electrical TF/1
  Voltage  saturation/1 -> Sum/1
  Electrical TF/1 -> Motor torque  constant/1
  Bias1/1 -> Product1/2, Product/1
  Product/1 -> Derivative/1
  Derivative/1 -> N_mw/1
  Product1/1 -> H_mw/1

== system components_lib/Actuator Emulation/NSO magnetorquers ==
  v_in : Inport  Port=1  LatchInput=off
  B(S) : Inport  Port=2  LatchInput=off
  T : Inport  Port=3  LatchInput=off
  Add : Sum  Inputs=+++  OutScaling=2^-10
  Demux : Demux  Outputs=3
  X Magnetorquer : components_lib/Actuator Emulation/Magnetorquer  v_max_mt=5  coil_dim=[0.07 0.21]  L_mt=26.956e-3  n_mt=435  A_wire_mt=(pi/4)*0.0002^2  sigma_0_mt=1.7e-8  alpha_0_mt=3.9e-3  T_0_mt=293
  X coil  normal : Constant  Value=[1;0;0]
  Y Magnetorquer : components_lib/Actuator Emulation/Magnetorquer  v_max_mt=5  coil_dim=[0.07 0.21]  L_mt=26.956e-3  n_mt=435  A_wire_mt=(pi/4)*0.0002^2  sigma_0_mt=1.7e-8  alpha_0_mt=3.9e-3  T_0_mt=293
  Y coil normal : Constant  Value=[0;1;0]
  Z Magnetorquer : components_lib/Actuator Emulation/Magnetorquer  v_max_mt=5  coil_dim=[0.07 0.07]  L_mt=59.256e-3  n_mt=865  A_wire_mt=(pi/4)*0.0002^2  sigma_0_mt=1.7e-8  alpha_0_mt=3.9e-3  T_0_mt=293
  Z coil normal : Constant  Value=[0;0;1]
  N_mt(S) : Outport  PortDimensions=3
  wires:
  v_in/1 -> Demux/1
  Add/1 -> N_mt(S)/1
  X coil  normal/1 -> X Magnetorquer/2
  Demux/1 -> X Magnetorquer/1
  X Magnetorquer/1 -> Add/1
  Y Magnetorquer/1 -> Add/2
  Z Magnetorquer/1 -> Add/3
  Demux/2 -> Y Magnetorquer/1
  Y coil normal/1 -> Y Magnetorquer/2
  Demux/3 -> Z Magnetorquer/1
  Z coil normal/1 -> Z Magnetorquer/2
  B(S)/1 -> Y Magnetorquer/3, X Magnetorquer/3, Z Magnetorquer/3
  T/1 -> Y Magnetorquer/4, X Magnetorquer/4, Z Magnetorquer/4

== system components_lib/Actuator Emulation/NSO magnetorquers without L ==
  v_in : Inport  Port=1  LatchInput=off
  B(S) : Inport  Port=2  LatchInput=off
  T : Inport  Port=3  LatchInput=off
  Add : Sum  Inputs=+++  OutScaling=2^-10
  Demux : Demux  Outputs=3
  "X Magnetorquer  without L " : components_lib/Actuator Emulation/Magnetorquer without L  v_max_mt=5  coil_dim=[0.07 0.21]  n_mt=435  A_wire_mt=(pi/4)*0.0002^2  sigma_0_mt=1.7e-8  alpha_0_mt=3.9e-3  T_0_mt=293
  X coil  normal : Constant  Value=[1;0;0]
  Y Magnetorquer  without L : components_lib/Actuator Emulation/Magnetorquer without L  v_max_mt=5  coil_dim=[0.07 0.21]  n_mt=435  A_wire_mt=(pi/4)*0.0002^2  sigma_0_mt=1.7e-8  alpha_0_mt=3.9e-3  T_0_mt=293
  Y coil normal : Constant  Value=[0;1;0]
  Z Magnetorquer  without L : components_lib/Actuator Emulation/Magnetorquer without L  v_max_mt=5  coil_dim=[0.07 0.07]  n_mt=865  A_wire_mt=(pi/4)*0.0002^2  sigma_0_mt=1.7e-8  alpha_0_mt=3.9e-3  T_0_mt=293
  Z coil normal : Constant  Value=[0;0;1]
  N_mt(S) : Outport  PortDimensions=3
  wires:
  T/1 -> "X Magnetorquer  without L "/4, Y Magnetorquer  without L/4, Z Magnetorquer  without L/4
  B(S)/1 -> "X Magnetorquer  without L "/3, Y Magnetorquer  without L/3, Z Magnetorquer  without L/3
  Z coil normal/1 -> Z Magnetorquer  without L/2
  Demux/3 -> Z Magnetorquer  without L/1
  Y coil normal/1 -> Y Magnetorquer  without L/2
  Demux/2 -> Y Magnetorquer  without L/1
  Z Magnetorquer  without L/1 -> Add/3
  Y Magnetorquer  without L/1 -> Add/2
  "X Magnetorquer  without L "/1 -> Add/1
  Demux/1 -> "X Magnetorquer  without L "/1
  X coil  normal/1 -> "X Magnetorquer  without L "/2
  Add/1 -> N_mt(S)/1
  v_in/1 -> Demux/1

== system components_lib/Actuator Emulation/NSO momentum wheels ==
  omega_ref : Inport  Port=1  LatchInput=off
  Add : Sum  Inputs=+++  OutScaling=2^-10
  Add1 : Sum  Inputs=+++  OutScaling=2^-10
  Add2 : Sum  Inputs=+++  OutScaling=2^-10
  Demux : Demux  Outputs=3
  Product{,1..5} (6 alike) : Product  RndMeth=Zero
  Produt1 : Product  RndMeth=Zero
  Produt2 : Product  RndMeth=Zero
  Produt6 : Product  RndMeth=Zero
  X Momentum wheel : components_lib/Actuator Emulation/NSO mw HW  C_p=0.4  C_i=0.04  w_mw_init=w_mw_i(1)
  X wheel : Constant  Value=[1;0;0]
  Y Momentum wheel : components_lib/Actuator Emulation/NSO mw HW  C_p=0.4  C_i=0.04  w_mw_init=w_mw_i(2)
  Y wheel : Constant  Value=[0;1;0]
  Z Momentum wheel : components_lib/Actuator Emulation/NSO mw HW  C_p=0.4  C_i=0.04  w_mw_init=w_mw_i(3)
  Z wheel : Constant  Value=[0;0;1]
  omega_mw : Outport  PortDimensions=3
  N_mw : Outport  Port=2  PortDimensions=3
  H_mw : Outport  Port=3  PortDimensions=3
  wires:
  Produt6/1 -> Add2/1
  Add2/1 -> H_mw/1
  Product1/1 -> Add1/1
  Product/1 -> Add/1
  Add1/1 -> N_mw/1
  X wheel/1 -> Product/2, Product1/2, Produt6/2
  Add/1 -> omega_mw/1
  X Momentum wheel/3 -> Produt6/1
  X Momentum wheel/1 -> Product/1
  X Momentum wheel/2 -> Product1/1
  Y wheel/1 -> Product2/2, Product3/2, Produt1/2
  Y Momentum wheel/3 -> Produt1/1
  Y Momentum wheel/1 -> Product2/1
  Y Momentum wheel/2 -> Product3/1
  Product2/1 -> Add/2
  Product3/1 -> Add1/2
  Produt1/1 -> Add2/2
  Z wheel/1 -> Product4/2, Product5/2, Produt2/2
  Z Momentum wheel/3 -> Produt2/1
  Z Momentum wheel/1 -> Product4/1
  Z Momentum wheel/2 -> Product5/1
  Produt2/1 -> Add2/3
  Product5/1 -> Add1/3
  Product4/1 -> Add/3
  omega_ref/1 -> Demux/1
  Demux/1 -> X Momentum wheel/1
  Demux/3 -> Z Momentum wheel/1
  Demux/2 -> Y Momentum wheel/1

== system components_lib/Actuator Emulation/NSO mw HW ==
  omega_ref : Inport  Port=1  LatchInput=off
  Momentum wheel : components_lib/Actuator Emulation/Momentum wheel  v_max_mw=3  v_min_mw=0  R_mw=8  L_mw=0.07e-3  C_t=2.67e-3  C_s=0.0027  mu_f=39.606e-9  I_mw=4.139e-6
  PI-controller : components_lib/Actuator Emulation/PI-controller  PI_cp=C_p  PI_ci=C_i  int_limit_max=3  int_limit_min=-3
  Sum3 : Sum  Inputs=-+|
  omega_mw : Outport  PortDimensions=1
  N_mw : Outport  Port=2  PortDimensions=1
  H_mw : Outport  Port=3  PortDimensions=1
  wires:
  omega_ref/1 -> Sum3/2
  Sum3/1 -> PI-controller/1
  PI-controller/1 -> Momentum wheel/1
  Momentum wheel/2 -> N_mw/1
  Momentum wheel/1 -> omega_mw/1, Sum3/1
  Momentum wheel/3 -> H_mw/1

== system components_lib/Actuator Emulation/PI-controller ==
  error signal : Inport  Port=1  LatchInput=off
  C_i : Gain  Gain=PI_ci
  C_p : Gain  Gain=PI_cp
  Integrator : Integrator  LimitOutput=on  UpperSaturationLimit=int_limit_max  LowerSaturationLimit=int_limit_min
  Sum : Sum  Inputs=+|+
  control signal : Outport
  wires:
  C_i/1 -> Sum/1
  C_p/1 -> Sum/2
  Integrator/1 -> C_i/1
  error signal/1 -> Integrator/1, C_p/1
  Sum/1 -> control signal/1

== system components_lib/Disturbances/Atmospheric ==
  q(I->S) : Inport  Port=1  LatchInput=off
  V_sc(I) : Inport  Port=2  LatchInput=off
  R_com(S) : Inport  Port=3  LatchInput=off
  Deployed : Inport  Port=4  LatchInput=off
  C_D : Constant  Value=Cd
  Density : Constant  Value=rho
  Dimensions : Constant  Value=Dim
  Exposed area : components_lib/Disturbances/Exposed area  dim_sat_area=Dim  dim_sat_array=[-0.30,-0.30]
  Gain : Gain  Gain=-1/2  SaturateOnIntegerOverflow=on
  Gain1 : Gain  Gain=1/2  SaturateOnIntegerOverflow=on
  Model Info : simulink/Model-Wide Utilities/Model Info  InitialBlockCM=None  BlockCM=None  Frame=on  DisplayStringWithTags=|  HorizontalTextAlignment=Center  LeftAlignmentValue=0.5  SourceBlockDiagram=components_lib  TagMaxNumber=20
      | The Constants Cd, 
      | rho and Dim are specified 
      | in the NSO mask
  Product{1..4} (4 alike) : Product  SaturateOnIntegerOverflow=on
  Sum : Sum  Inputs=|-+
  Vector rotation by q : components_lib/Math utilities/Vector operations/Vector rotation by q
  cross_product_no_fnc : components_lib/Math utilities/Vector operations/cross_product_no_fnc
  math operation : Math  Operator=magnitude^2  SaturateOnIntegerOverflow=on
  to unit vector : components_lib/Math utilities/Vector operations/to unit vector
  N_atm(S) : Outport
  F_atm(I) : Outport  Port=2
  wires:
  Sum/1 -> cross_product_no_fnc/1
  R_com(S)/1 -> Sum/1  "Center of Mass"
  Gain1/1 -> Sum/2  "Geometric Center"
  Dimensions/1 -> Gain1/1
  Vector rotation by q/1 -> cross_product_no_fnc/2
  Gain/1 -> F_atm(I)/1, Vector rotation by q/2
  Product4/1 -> Gain/1
  q(I->S)/1 -> Vector rotation by q/1, Exposed area/1
  Density/1 -> Product3/2
  Product2/1 -> Product3/1
  Product1/1 -> Product2/2
  math operation/1 -> Product1/1
  to unit vector/1 -> Product1/2
  V_sc(I)/1 -> to unit vector/1, math operation/1, Exposed area/2
  Exposed area/1 -> Product2/1
  C_D/1 -> Product4/1
  Product3/1 -> Product4/2
  cross_product_no_fnc/1 -> N_atm(S)/1
  Deployed/1 -> Exposed area/3

== system components_lib/Disturbances/Disturbances ==
  Moon positon R_m(I) : Inport  Port=1  LatchInput=off
  Sun position R_s(I) : Inport  Port=2  LatchInput=off
  Inertia folded I_f(C) : Inport  Port=3  LatchInput=off
  Orbit position R_sc(I) : Inport  Port=4  LatchInput=off
  "Attitude q(I -> SC)" : Inport  Port=5  LatchInput=off
  Orbit velocity V_sc(I) : Inport  Port=6  LatchInput=off
  Center of mass  R_com(SC) : Inport  Port=7  LatchInput=off
  "Mass of Spacecraft " : Inport  Port=8  LatchInput=off
  q(SC->C) : Inport  Port=9  LatchInput=off
  eclipse : Inport  Port=10  LatchInput=off
  Inertia deployed I_d(C) : Inport  Port=11  LatchInput=off
  deployed : Inport  Port=12  LatchInput=off
  R_com_deployed : Inport  Port=13  LatchInput=off
  Atmospheric : components_lib/Disturbances/Atmospheric
  Gravity : components_lib/Disturbances/Gravity  G=6.673e-11  M_sun=1.98892e30  M_moon=7.36e22  M_earth=5.9742e24
  Quaternion inverter : components_lib/Math utilities/Quaternion operations/Quaternion inverter
  Radiation (I) : components_lib/Disturbances/Radiation (I)
  Sum1 : Sum  Inputs=+++  SaturateOnIntegerOverflow=on
  Sum2 : Sum  Inputs=+++  SaturateOnIntegerOverflow=on
  Switch : Switch  Criteria=u2 > Threshold
  Switch1 : Switch  Criteria=u2 > Threshold
  Disturbance tourque N_dist(sc) : Outport
  Disturbance Force F_dist(I) : Outport  Port=2
  wires:
  Switch1/1 -> Atmospheric/3, Radiation (I)/4
  R_com_deployed/1 -> Switch1/1
  Center of mass  R_com(SC)/1 -> Switch1/3
  q(SC->C)/1 -> Quaternion inverter/1
  Quaternion inverter/1 -> Gravity/6
  "Mass of Spacecraft "/1 -> Gravity/7
  Moon positon R_m(I)/1 -> Gravity/1  "R_m(I)"
  Sun position R_s(I)/1 -> Gravity/2, Radiation (I)/1  "R_s(I)"
  "Attitude q(I -> SC)"/1 -> Atmospheric/1, Radiation (I)/3, Gravity/5
  Orbit position R_sc(I)/1 -> Gravity/3, Radiation (I)/2
  Orbit velocity V_sc(I)/1 -> Atmospheric/2
  Radiation (I)/1 -> Sum1/1
  Atmospheric/1 -> Sum1/2
  Gravity/1 -> Sum1/3
  Radiation (I)/2 -> Sum2/1
  Atmospheric/2 -> Sum2/2
  Gravity/2 -> Sum2/3
  Sum1/1 -> Disturbance tourque N_dist(sc)/1
  Sum2/1 -> Disturbance Force F_dist(I)/1
  eclipse/1 -> Radiation (I)/5
  Inertia folded I_f(C)/1 -> Switch/3
  Inertia deployed I_d(C)/1 -> Switch/1
  Switch/1 -> Gravity/4
  deployed/1 -> Switch1/2, Switch/2, Atmospheric/4, Radiation (I)/6

== system components_lib/Disturbances/Exposed area ==
  quaternion : Inport  Port=1  LatchInput=off
  vector : Inport  Port=2  LatchInput=off
  deployed : Inport  Port=3  LatchInput=off
  Product{2..6} (5 alike) : Product  Multiplication=Matrix(*)  RndMeth=Zero
  Projection Matrix1 : Subsystem
  Satellite Area : Subsystem
  Shadow Area : Subsystem
  Solar Array Area : Subsystem
  Sum1 : Sum  Inputs=+|-|+
  Switch : Switch  Criteria=u2 ~= 0
  Vector rotation by q3 : components_lib/Math utilities/Quaternion operations/Vector rotation by q
  f1_y : Constant  Value=[0 dim_sat_array(1) 0]'
  f2_x : Constant  Value=[dim_sat_array(2) 0 0]'
  to unit vector4 : components_lib/Math utilities/Vector operations/to unit vector
  x : Constant  Value=[dim_sat_area(1) 0 0]'
  y : Constant  Value=[0 dim_sat_area(2) 0]'
  z : Constant  Value=[0 0 dim_sat_area(3)]'
  exposed area : Outport
  wires:
  deployed/1 -> Switch/2
  Switch/1 -> exposed area/1
  Vector rotation by q3/1 -> Projection Matrix1/1(n-vector)
  Sum1/1 -> Switch/1
  Solar Array Area/1(area_flaps) -> Sum1/3
  Shadow Area/1(area_shadow) -> Sum1/2
  Satellite Area/1(area_sat) -> Switch/3, Sum1/1
  Product6/1 -> Solar Array Area/4(f2_px), Shadow Area/5(f2_px)
  Product5/1 -> Shadow Area/4(f1_py), Solar Array Area/1(f1_py)
  Product3/1 -> Shadow Area/3(pz), Satellite Area/3(pz)
  Product4/1 -> Solar Array Area/3(py), Shadow Area/2(py), Satellite Area/2(py)
  Product2/1 -> Solar Array Area/2(px), Shadow Area/1(px), Satellite Area/1(px)
  f2_x/1 -> Product6/2
  f1_y/1 -> Product5/2
  z/1 -> Product3/2
  y/1 -> Product4/2
  x/1 -> Product2/2
  Projection Matrix1/1(P matrix) -> Product6/1, Product5/1, Product3/1, Product4/1, Product2/1
  quaternion/1 -> Vector rotation by q3/1
  vector/1 -> to unit vector4/1
  to unit vector4/1 -> Vector rotation by q3/2
